simulink model "e5_2nd"  (R2016b)
settings: Solver=VariableStepAuto  StartTime=0.0  StopTime=2  RelTol=1e-3
values from neighbouring files (symbols this model uses):
  A = ones(5 ,7)    [Exp_1.m]    (also in Q7.m = [1 1 0 1 0 ; 0 -1 1 0 1 ])
  Torque = 0:50:500    [dcmotor.m]
libraries: powerlib x9
settings Model: Creator=hp  LastModifiedBy=hp

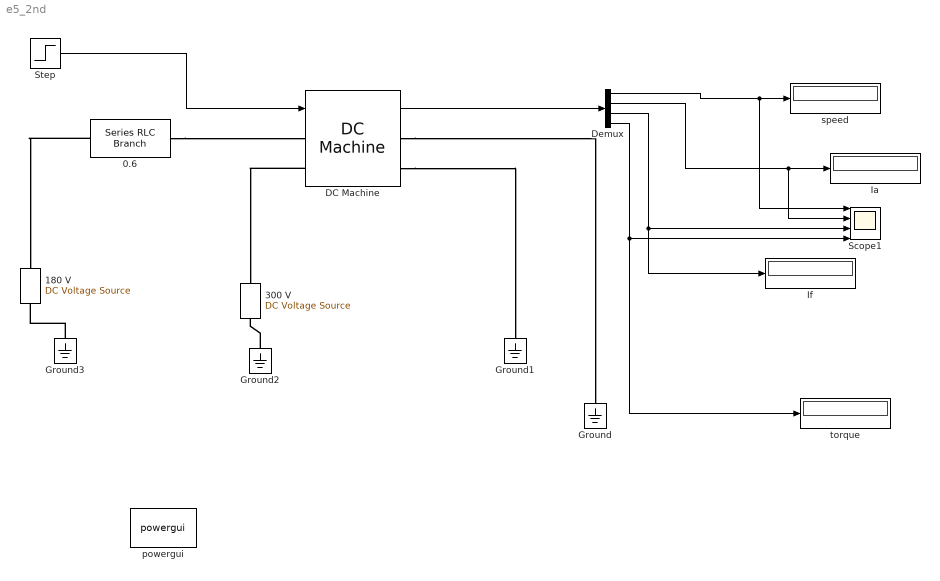
== system e5_2nd ==
  "0.6 " : powerlib/Elements/Series RLC Branch  LConnTagsString=__new0  RConnTagsString=__new0  BranchType=R  Resistance=0.6  Inductance=1e-3  SetiL0=off  InitialCurrent=0  Capacitance=1e-6  Setx0=off  InitialVoltage=0  Measurements=None
  "180 V " : powerlib/Electrical Sources/DC Voltage Source  Amplitude=180  Measurements=None
  300 V : powerlib/Electrical Sources/DC Voltage Source  Amplitude=300  Measurements=None
  DC Machine : powerlib/Machines/DC Machine  PresetModel=No  MechanicalLoad=Torque TL  FieldType=Wound  ShowDetailedParameters=on  MeasurementBus=off  RLa="[ 0.6  0.012]"  RLf="[ 240  120]"  Laf=1.8  MachineConstant=Torque constant (N.m/A)  Ke=1.8  Kt=1.8  J=1  Bm=0  Tf=0  w0=1  Ifinit=1  TsPowergui=0  TsBlock=-1
  Demux : Demux
  Ground{,1..3} (4 alike) : powerlib/Elements/Ground  LConnTagsString=a
  Ia : Display
  If : Display
  Scope1 : Scope  NumInputPorts=4
  Step : Step  SampleTime=0
  powergui : powerlib/powergui  Priority=1  SimulationMode=Continuous  SolverType=Tustin/Backward Euler (TBE)  SampleTime=50e-6  frequency=60  SPID=off  DisableSnubberDevices=off  DisableRonSwitches=off  DisableVfSwitches=off  SwTol=0  DisplayEquations=off  Interpol=off  ExternalGateDelay=off  methode=off  Ts=10  FunctionMessages=off  echomessages=off  HookPort=off  EnableUseOfTLC=off  x0status=blocks  frequencyindice=0  Pbase=100e6  ErrMax=1e-4  Iterations=50  UnitsV=kV  UnitsW=MW  buscounter=0  RestoreLinks=warning  ResistiveCurrentMeasurement=off  Frange=[0:2:500]  Ylog=off  Xlog=on  ShowGrid=off  save=off  variable=ZData  structure=0  ZoomFFT=off  StartTime=0.0  cycles=1  DisplayStyle=1  fundamental=60  FreqAxis=off  MaxFrequency=1000  frequencyindicesteady=1  RmsSteady=1  display=off
  "speed " : Display
  "torque " : Display
  wires:
  DC Machine/1 -> Demux/1
  Step/1 -> DC Machine/1
  Demux/1 -> Scope1/1, "speed "/1
  Demux/2 -> Scope1/2, Ia/1
  Demux/3 -> Scope1/3, If/1
  Demux/4 -> Scope1/4, "torque "/1
  connections:
  Ground2/LConn1 -- 300 V/LConn1
  DC Machine/RConn1 -- Ground/LConn1
  Ground3/LConn1 -- "180 V "/LConn1
  "0.6 "/LConn1 -- "180 V "/RConn1
  "0.6 "/RConn1 -- DC Machine/LConn1
  DC Machine/LConn2 -- 300 V/RConn1
  DC Machine/RConn2 -- Ground1/LConn1
